simulink model "receiver"  (R2021b)
settings: Solver=VariableStepAuto  StartTime=0.0  StopTime=30  RelTol=1e-3
settings Model: DataDictionary=can_messaging.sldd  Creator=grodriguez  LastModifiedBy=vgaggero

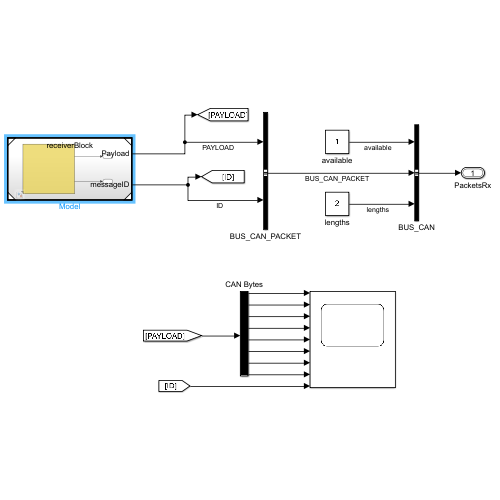
[thumbnail: Simulink's stored preview of the top-level diagram]
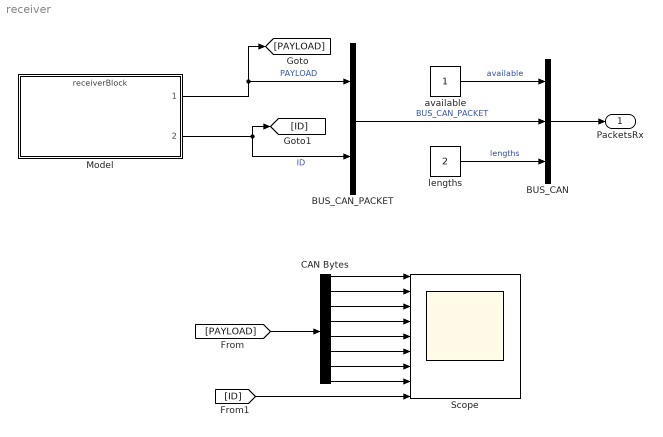
== system receiver ==
  BUS_CAN : BusCreator  Inputs=3
  BUS_CAN_PACKET : BusCreator  Inputs=2
  CAN Bytes : Demux  Outputs=8
  Model : ModelReference  ModelNameDialog=receiverBlock.slx  SimulationMode=Normal  ModelReferenceVersion=1.4
  Scope : Scope  NumInputPorts=9
  available : Constant
  lengths : Constant  Value=2
  PacketsRx : Outport  OutDataTypeStr=Bus: BUS_CAN
  wires:
  Model/1 -> [PAYLOAD], BUS_CAN_PACKET/1  "PAYLOAD"
  CAN Bytes/1 -> Scope/1
  CAN Bytes/2 -> Scope/2
  CAN Bytes/3 -> Scope/3
  CAN Bytes/4 -> Scope/4
  CAN Bytes/5 -> Scope/5
  CAN Bytes/6 -> Scope/6
  CAN Bytes/7 -> Scope/7
  CAN Bytes/8 -> Scope/8
  Model/2 -> BUS_CAN_PACKET/2, [ID]  "ID"
  available/1 -> BUS_CAN/1  "available"
  lengths/1 -> BUS_CAN/3  "lengths"
  BUS_CAN_PACKET/1 -> BUS_CAN/2  "BUS_CAN_PACKET"
  BUS_CAN/1 -> PacketsRx/1
  [PAYLOAD] -> CAN Bytes/1
  [ID] -> Scope/9
